simulink model "Mil_Light"  (R2020b)
settings: Solver=VariableStepAuto  StartTime=0.0  StopTime=10.0  RelTol=1e-3
undefined symbols (not defined in the file): sigbuilder_block
settings Model: Creator=training  LastModifiedBy=training

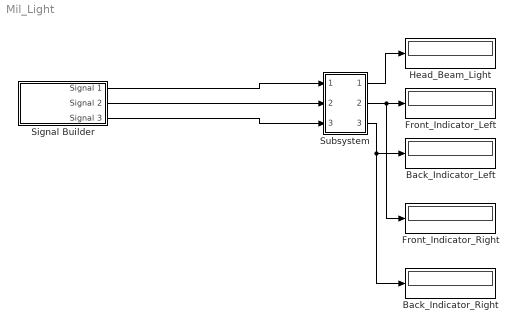
== system Mil_Light ==
  Back_Indicator_Left : Display
  Back_Indicator_Right : Display
  Front_Indicator_Left : Display
  Front_Indicator_Right : Display
  Head_Beam_Light : Display
  Signal Builder : Subsystem  Tag=STV Subsys  LoadFcn=sigbuilder_block('load');  StartFcn=sigbuilder_block('start');  StopFcn=sigbuilder_block('stop');  ClipboardFcn=sigbuilder_block('clipboard');  mask(Sigbuilder block){tuvar=[0:10]}
      mask help: Simulink:masks:SigbuilderBlock_MD
      mask init:
      | if ~strcmp(get_param(bdroot(gcbh),'SimulationStatus'),'stopped') tuvar = sigbuilder_block('maskInit'); end
      settings: CopyFcn=sigbuilder_block('copy');  DeleteFcn=sigbuilder_block('delete');  ModelCloseFcn=sigbuilder_block('modelClose');  PreSaveFcn=sigbuilder_block('preSave');  PauseFcn=sigbuilder_block('pause');  ContinueFcn=sigbuilder_block('continue');  NameChangeFcn=sigbuilder_block('namechange');  OpenFcn=sigbuilder_block('open',[437.6 153 550.4 359.25 ]);  CloseFcn=sigbuilder_block('close');
      mask Display: plot(0, 0, 100, 100,[2, 2, 32, 32, 2], [68, 8, 8, 68, 68],[32, 2], [38, 38], [32, 19, 2],[53, 60, 44], [32, 17, 17, 2],[16, 16, 31, 31]);txt = getActiveGroup(gcbh);text(2, 100, txt,'verticalAlignment', 'top');
  Subsystem : Subsystem
  wires:
  Signal Builder/1(Signal 1) -> Subsystem/1(In1)
  Signal Builder/2(Signal 2) -> Subsystem/2(In2)
  Subsystem/1(Out1) -> Head_Beam_Light/1
  Subsystem/2(Out2) -> Front_Indicator_Right/1, Front_Indicator_Left/1
  Subsystem/3(Out3) -> Back_Indicator_Right/1, Back_Indicator_Left/1
  Signal Builder/3(Signal 3) -> Subsystem/3(In3)

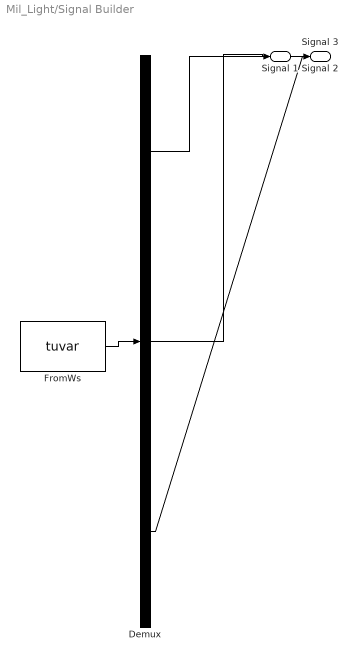
== system Mil_Light/Signal Builder ==
  Demux : Demux  Tag=STV Demux  Outputs=3
      settings: DisplayOption=none
  FromWs : FromWorkspace  Tag=STV FromWs  VariableName=tuvar
      SigBuilderData=|
      | common.afterFinalStr = 'Extrapolate'
      | common.sampleTime = 0
      | dataSet.timeRange = [0 10]
      | dataSet.name = 'Group 1'
      | sbobj.Groups.Name = 'Group 1'
      | sbobj.Groups.Signals(1).Name = 'Signal 1'
      | sbobj.Groups.Signals(1).XData = [0 4 4 6 6 10]
      | sbobj.Groups.Signals(1).YData = [0 0 1 1 0 0]
      | sbobj.Groups.Signals(2).Name = 'Signal 2'
      | sbobj.Groups.Signals(2).XData = [0 1 1 2 2 3 3 4 4 5 5 6 6 7 7 8 8 9 9 10]
      | sbobj.Groups.Signals(2).YData = [0 2 0 2 0 2 0 2 0 2 0 2 0 2 0 2 0 2 0 2]
      | sbobj.Groups.Signals(3).Name = 'Signal 3'
      | sbobj.Groups.Signals(3).XData = [0 0.5 0.5 1 1 1.5 1.5 2 2 2.5 2.5 3 3 3.5 3.5 4 4 4.5 4.5 5 5 5.5 5.5 6 6 6.5 6.5 7 7 7.5 7.5 8 8 8.5 8.5 9 9 9.5 9.5 10]
      | sbobj.Groups.Signals(3).YData = [2 2 0 0 2 2 0 0 2 2 0 0 2 2 0 0 2 2 0 0 2 2 0 0 2 2 0 0 2 2 0 0 2 2 0 0 2 2 0 0]
  Signal 1 : Outport  Tag=STV Outport
  Signal 2 : Outport  Tag=STV Outport  Port=2
  Signal 3 : Outport  Tag=STV Outport  Port=3
  wires:
  Demux/1 -> Signal 1/1
  FromWs/1 -> Demux/1
  Demux/2 -> Signal 2/1
  Demux/3 -> Signal 3/1

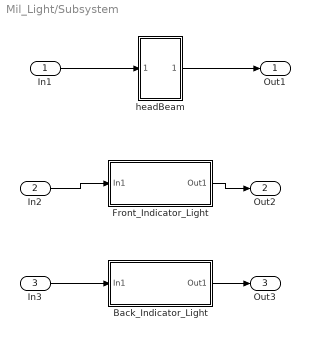
== system Mil_Light/Subsystem ==
  In1 : Inport
  In2 : Inport  Port=2
  In3 : Inport  Port=3
  Back_Indicator_Light : Subsystem  Variant=on
  Front_Indicator_Light : Subsystem  Variant=on
  headBeam : Subsystem
  Out1 : Outport
  Out2 : Outport  Port=2
  Out3 : Outport  Port=3
  wires:
  Back_Indicator_Light/1(Out1) -> Out3/1
  In1/1 -> headBeam/1(In1)
  In2/1 -> Front_Indicator_Light/1(In1)
  Front_Indicator_Light/1(Out1) -> Out2/1
  headBeam/1(Out1) -> Out1/1
  In3/1 -> Back_Indicator_Light/1(In1)

== system Mil_Light/Subsystem/Back_Indicator_Light ==
  note: 1) Add Subsystem or Model blocks as valid variant choices.
      | 2) You cannot connect blocks at this level. At simulation, connectivity is automatically
      | determined, based on the active variant and port name matching.
  In1 : Inport
  Back_Indicator_Left : Subsystem  VariantControl=Choice_1
  Back_Indicator_Right : Subsystem  VariantControl=Choice_2
  Out1 : Outport

== system Mil_Light/Subsystem/Front_Indicator_Light ==
  note: 1) Add Subsystem or Model blocks as valid variant choices.
      | 2) You cannot connect blocks at this level. At simulation, connectivity is automatically
      | determined, based on the active variant and port name matching.
  In1 : Inport
  Front_Indicator_Left : Subsystem  VariantControl=Choice_1
  Front_Indicator_Right : Subsystem  VariantControl=Choice_2
  Out1 : Outport

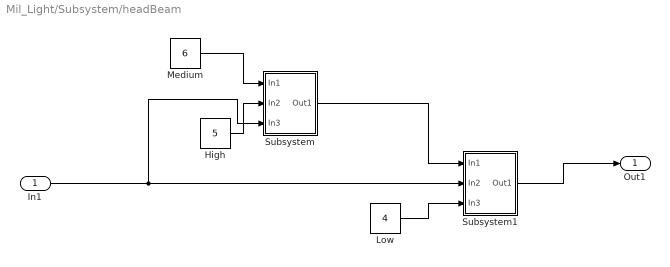
== system Mil_Light/Subsystem/headBeam ==
  In1 : Inport
  High : Constant  Value=5
  Low : Constant  Value=4
  Medium : Constant  Value=6
  Subsystem : Subsystem
  Subsystem1 : Subsystem
  Out1 : Outport
  wires:
  High/1 -> Subsystem/2(In2)
  Subsystem/1(Out1) -> Subsystem1/1(In1)
  Medium/1 -> Subsystem/1(In1)
  In1/1 -> Subsystem/3(In3), Subsystem1/2(In2)
  Low/1 -> Subsystem1/3(In3)
  Subsystem1/1(Out1) -> Out1/1

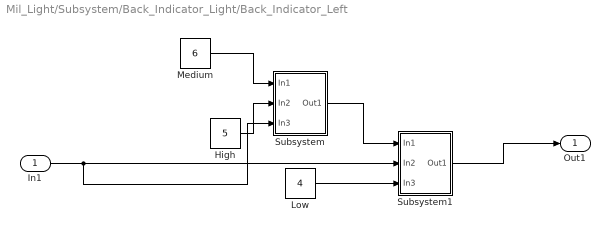
== system Mil_Light/Subsystem/Back_Indicator_Light/Back_Indicator_Left ==
  In1 : Inport
  High : Constant  Value=5
  Low : Constant  Value=4
  Medium : Constant  Value=6
  Subsystem : Subsystem
  Subsystem1 : Subsystem
  Out1 : Outport
  wires:
  In1/1 -> Subsystem/3(In3), Subsystem1/2(In2)
  Subsystem1/1(Out1) -> Out1/1
  Subsystem/1(Out1) -> Subsystem1/1(In1)
  High/1 -> Subsystem/2(In2)
  Medium/1 -> Subsystem/1(In1)
  Low/1 -> Subsystem1/3(In3)

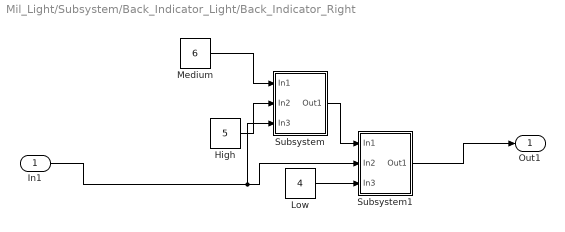
== system Mil_Light/Subsystem/Back_Indicator_Light/Back_Indicator_Right ==
  In1 : Inport
  High : Constant  Value=5
  Low : Constant  Value=4
  Medium : Constant  Value=6
  Subsystem : Subsystem
  Subsystem1 : Subsystem
  Out1 : Outport
  wires:
  Low/1 -> Subsystem1/3(In3)
  Subsystem/1(Out1) -> Subsystem1/1(In1)
  High/1 -> Subsystem/2(In2)
  In1/1 -> Subsystem/3(In3), Subsystem1/2(In2)
  Subsystem1/1(Out1) -> Out1/1
  Medium/1 -> Subsystem/1(In1)

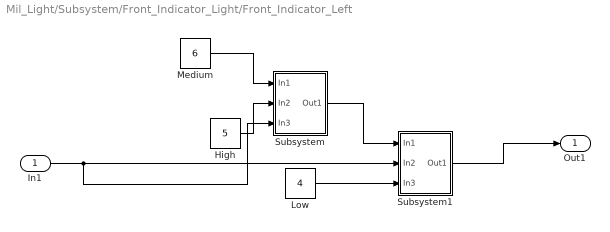
== system Mil_Light/Subsystem/Front_Indicator_Light/Front_Indicator_Left ==
  In1 : Inport
  High : Constant  Value=5
  Low : Constant  Value=4
  Medium : Constant  Value=6
  Subsystem : Subsystem
  Subsystem1 : Subsystem
  Out1 : Outport
  wires:
  In1/1 -> Subsystem/3(In3), Subsystem1/2(In2)
  Subsystem1/1(Out1) -> Out1/1
  Subsystem/1(Out1) -> Subsystem1/1(In1)
  High/1 -> Subsystem/2(In2)
  Medium/1 -> Subsystem/1(In1)
  Low/1 -> Subsystem1/3(In3)

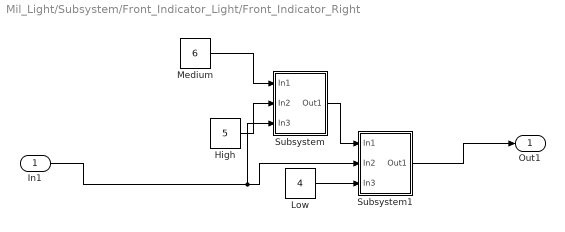
== system Mil_Light/Subsystem/Front_Indicator_Light/Front_Indicator_Right ==
  In1 : Inport
  High : Constant  Value=5
  Low : Constant  Value=4
  Medium : Constant  Value=6
  Subsystem : Subsystem
  Subsystem1 : Subsystem
  Out1 : Outport
  wires:
  Low/1 -> Subsystem1/3(In3)
  Subsystem/1(Out1) -> Subsystem1/1(In1)
  High/1 -> Subsystem/2(In2)
  In1/1 -> Subsystem/3(In3), Subsystem1/2(In2)
  Subsystem1/1(Out1) -> Out1/1
  Medium/1 -> Subsystem/1(In1)

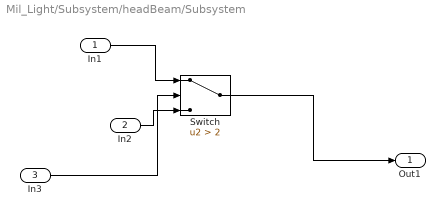
== system Mil_Light/Subsystem/headBeam/Subsystem ==
  In1 : Inport
  In2 : Inport  Port=2
  In3 : Inport  Port=3
  Switch : Switch  Criteria=u2 > Threshold  Threshold=2
  Out1 : Outport
  wires:
  In3/1 -> Switch/2
  Switch/1 -> Out1/1
  In1/1 -> Switch/1
  In2/1 -> Switch/3

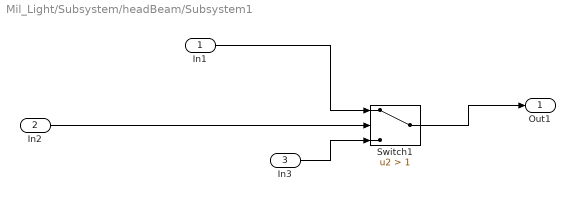
== system Mil_Light/Subsystem/headBeam/Subsystem1 ==
  In1 : Inport
  In2 : Inport  Port=2
  In3 : Inport  Port=3
  Switch1 : Switch  Criteria=u2 > Threshold  Threshold=1
  Out1 : Outport
  wires:
  In1/1 -> Switch1/1
  Switch1/1 -> Out1/1
  In3/1 -> Switch1/3
  In2/1 -> Switch1/2

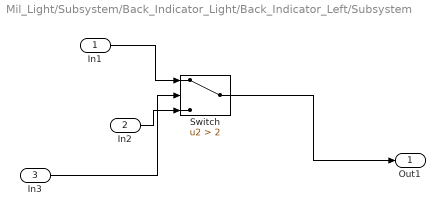
== system Mil_Light/Subsystem/Back_Indicator_Light/Back_Indicator_Left/Subsystem ==
  In1 : Inport
  In2 : Inport  Port=2
  In3 : Inport  Port=3
  Switch : Switch  Criteria=u2 > Threshold  Threshold=2
  Out1 : Outport
  wires:
  In3/1 -> Switch/2
  Switch/1 -> Out1/1
  In1/1 -> Switch/1
  In2/1 -> Switch/3

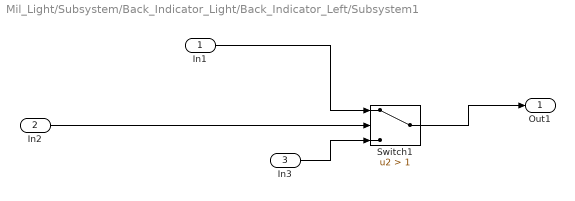
== system Mil_Light/Subsystem/Back_Indicator_Light/Back_Indicator_Left/Subsystem1 ==
  In1 : Inport
  In2 : Inport  Port=2
  In3 : Inport  Port=3
  Switch1 : Switch  Criteria=u2 > Threshold  Threshold=1
  Out1 : Outport
  wires:
  In1/1 -> Switch1/1
  Switch1/1 -> Out1/1
  In3/1 -> Switch1/3
  In2/1 -> Switch1/2

== system Mil_Light/Subsystem/Back_Indicator_Light/Back_Indicator_Right/Subsystem ==
  In1 : Inport
  In2 : Inport  Port=2
  In3 : Inport  Port=3
  Switch : Switch  Criteria=u2 > Threshold  Threshold=2
  Out1 : Outport
  wires:
  In3/1 -> Switch/2
  Switch/1 -> Out1/1
  In1/1 -> Switch/1
  In2/1 -> Switch/3

== system Mil_Light/Subsystem/Back_Indicator_Light/Back_Indicator_Right/Subsystem1 ==
  In1 : Inport
  In2 : Inport  Port=2
  In3 : Inport  Port=3
  Switch1 : Switch  Criteria=u2 > Threshold  Threshold=1
  Out1 : Outport
  wires:
  In1/1 -> Switch1/1
  Switch1/1 -> Out1/1
  In3/1 -> Switch1/3
  In2/1 -> Switch1/2

== system Mil_Light/Subsystem/Front_Indicator_Light/Front_Indicator_Left/Subsystem ==
  In1 : Inport
  In2 : Inport  Port=2
  In3 : Inport  Port=3
  Switch : Switch  Criteria=u2 > Threshold  Threshold=2
  Out1 : Outport
  wires:
  In3/1 -> Switch/2
  Switch/1 -> Out1/1
  In1/1 -> Switch/1
  In2/1 -> Switch/3

== system Mil_Light/Subsystem/Front_Indicator_Light/Front_Indicator_Left/Subsystem1 ==
  In1 : Inport
  In2 : Inport  Port=2
  In3 : Inport  Port=3
  Switch1 : Switch  Criteria=u2 > Threshold  Threshold=1
  Out1 : Outport
  wires:
  In1/1 -> Switch1/1
  Switch1/1 -> Out1/1
  In3/1 -> Switch1/3
  In2/1 -> Switch1/2

== system Mil_Light/Subsystem/Front_Indicator_Light/Front_Indicator_Right/Subsystem ==
  In1 : Inport
  In2 : Inport  Port=2
  In3 : Inport  Port=3
  Switch : Switch  Criteria=u2 > Threshold  Threshold=2
  Out1 : Outport
  wires:
  In3/1 -> Switch/2
  Switch/1 -> Out1/1
  In1/1 -> Switch/1
  In2/1 -> Switch/3

== system Mil_Light/Subsystem/Front_Indicator_Light/Front_Indicator_Right/Subsystem1 ==
  In1 : Inport
  In2 : Inport  Port=2
  In3 : Inport  Port=3
  Switch1 : Switch  Criteria=u2 > Threshold  Threshold=1
  Out1 : Outport
  wires:
  In1/1 -> Switch1/1
  Switch1/1 -> Out1/1
  In3/1 -> Switch1/3
  In2/1 -> Switch1/2
